simulink model "M3d"  (R2021b)
settings: Solver=ode45  StartTime=0.0  StopTime=10.0  MaxStep=0.01  RelTol=1e-3
settings Model: Creator=Studenci  LastModifiedBy=Studenci

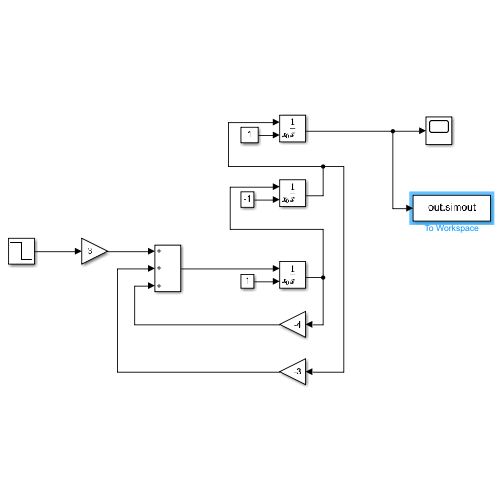
[thumbnail: Simulink's stored preview of the top-level diagram]
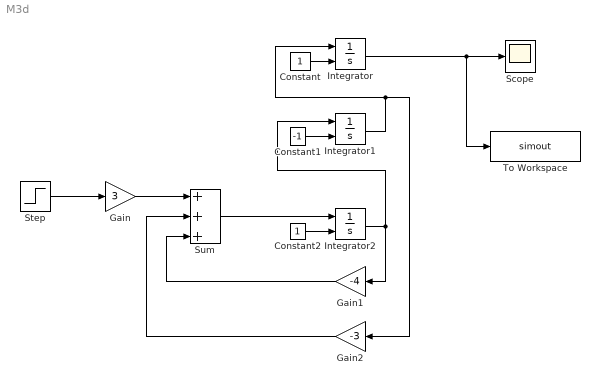
== system M3d ==
  Constant : Constant
  Constant1 : Constant  Value=-1
  Constant2 : Constant
  Gain : Gain  Gain=3
  Gain1 : Gain  Gain=-4
  Gain2 : Gain  Gain=-3
  Integrator : Integrator  InitialConditionSource=external
  Integrator1 : Integrator  InitialConditionSource=external
  Integrator2 : Integrator  InitialConditionSource=external
  Scope : Scope
  Step : Step  Time=0.01  Before=100  After=0  SampleTime=0
  Sum : Sum  Inputs=+++
  To Workspace : ToWorkspace  VariableName=simout  SaveFormat=Timeseries  SampleTime=-1
  wires:
  Constant/1 -> Integrator/2
  Constant2/1 -> Integrator2/2
  Constant1/1 -> Integrator1/2
  Sum/1 -> Integrator2/1
  Integrator2/1 -> Gain1/1, Integrator1/1
  Integrator1/1 -> Gain2/1, Integrator/1
  Integrator/1 -> To Workspace/1, Scope/1
  Step/1 -> Gain/1
  Gain1/1 -> Sum/3
  Gain2/1 -> Sum/2
  Gain/1 -> Sum/1
